simulink library "DP"  (Simulink 8.1)
settings: Solver=ode3  StartTime=0.0  StopTime=10.0  RelTol=1e-3
undefined symbols (not defined in the file): Dcontrol, Icontrol, Pcontrol, Thrust0, x_ref
settings Model: Creator=torstebo  LastModifiedBy=torstebo

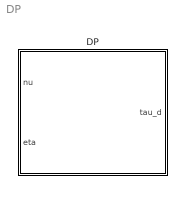
== system DP ==
  DP : Subsystem

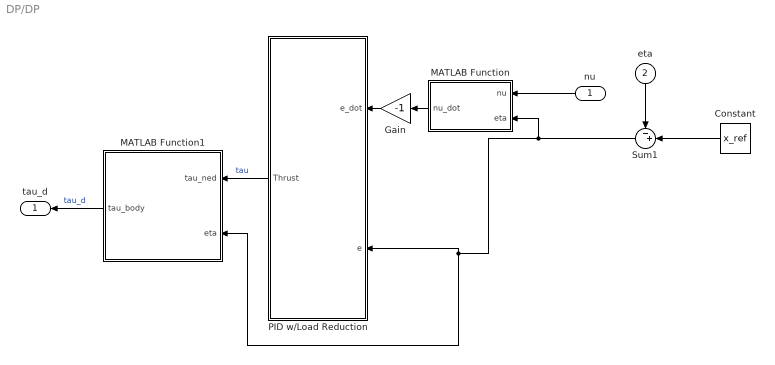
== system DP/DP ==
  nu : Inport
  eta : Inport  Port=2
  Constant : Constant  Value=x_ref
  Gain : Gain  Gain=-1
  MATLAB Function : MATLAB Function  TreatAsAtomicUnit=on
  MATLAB Function1 : MATLAB Function  TreatAsAtomicUnit=on
  PID w/Load Reduction : Subsystem
  Sum1 : Sum  Inputs=-+|
  tau_d : Outport
  wires:
  nu/1 -> MATLAB Function/1(nu)
  Gain/1 -> PID w/Load Reduction/1(e_dot)
  Constant/1 -> Sum1/2
  eta/1 -> Sum1/1
  Sum1/1 -> MATLAB Function/2(eta), MATLAB Function1/2(eta), PID w/Load Reduction/2(e)
  MATLAB Function/1(nu_dot) -> Gain/1
  MATLAB Function1/1(tau_body) -> tau_d/1  "tau_d"
  PID w/Load Reduction/1(Thrust) -> MATLAB Function1/1(tau_ned)  "tau"

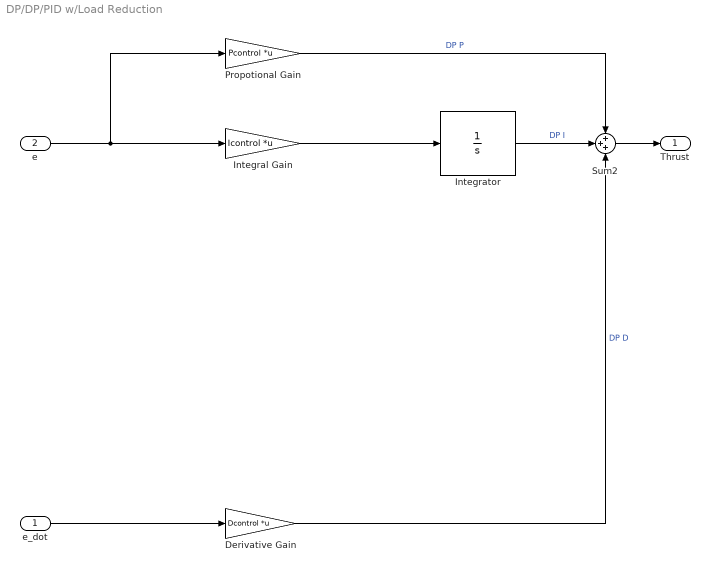
== system DP/DP/PID w/Load Reduction ==
  e_dot : Inport
  e : Inport  Port=2
  Derivative Gain : Gain  Gain=Dcontrol  Multiplication=Matrix(K*u)
  Integral Gain : Gain  Gain=Icontrol  Multiplication=Matrix(K*u)
  Integrator : Integrator  InitialCondition=Thrust0  ZeroCross=off
  Propotional Gain : Gain  Gain=Pcontrol  Multiplication=Matrix(K*u)
  Sum2 : Sum  Inputs=+++
  Thrust : Outport
  wires:
  e/1 -> Propotional Gain/1, Integral Gain/1
  Integrator/1 -> Sum2/2  "DP I"
  Sum2/1 -> Thrust/1
  e_dot/1 -> Derivative Gain/1
  Derivative Gain/1 -> Sum2/3  "DP D"
  Propotional Gain/1 -> Sum2/1  "DP P"
  Integral Gain/1 -> Integrator/1

== matlab function DP/MATLAB Function ==
  data: nu input double; nu_dot output double; eta input double
function nu_dot = rotateBody2Ned(nu,eta)
%#codegen
psi = eta(3);

nu_dot = [cos(psi) -sin(psi) 0
    sin(psi)    cos(psi)    0
    0   0   1]*nu;

== matlab function DP/MATLAB Function1 ==
  data: tau_ned input double; tau_body output double; eta input double
function tau_body = rotateNed2Body(tau_ned,eta)
%#codegen
psi = eta(3);

tau_body = [cos(psi) sin(psi) 0
    -sin(psi)    cos(psi)    0
    0   0   1]*tau_ned;
